simulink model "TrajGen"  (R2015a)
settings: Solver=ode45  StartTime=0.0  StopTime=10.0  RelTol=1e-3
values from neighbouring files (symbols this model uses):
  hf = 0    [ConvertToTimeseries.m]    (also in createTrajectories.m = -90)
  hi = 0    [ConvertToTimeseries.m]    (also in createTrajectories.m = 20)
  l = 10    [ConvertToTimeseries.m]    (also in createTrajectories.m = 3)
  xf = 63.37    [ConvertToTimeseries.m]    (also in createTrajectories.m = -5; genTraj.m = FC(1:3))
  xi = -10.89    [ConvertToTimeseries.m]    (also in createTrajectories.m = -6; genTraj.m = IC(1:3))
  yf = 48.737    [ConvertToTimeseries.m]    (also in createTrajectories.m = -6)
  yi = 48.737    [ConvertToTimeseries.m]    (also in createTrajectories.m = 2)
  zf = 2.33    [ConvertToTimeseries.m]    (also in createTrajectories.m = 2)
  zi = 2.33    [ConvertToTimeseries.m]    (also in createTrajectories.m = 2)
libraries: simulink x1
settings Model: CovSFcnEnable=off  Creator=cichell2  LastModifiedBy=marinho
settings DebuggingCC: SolverPrmCheckMsg=warning

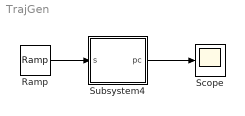
== system TrajGen ==
  Ramp : simulink/Sources/Ramp  slope=0.1  start=0  X0=0
  Scope : Scope
      settings: SaveName=Trajectory
  Subsystem4 : Subsystem
  wires:
  Ramp/1 -> Subsystem4/1(s)
  Subsystem4/1(pc) -> Scope/1

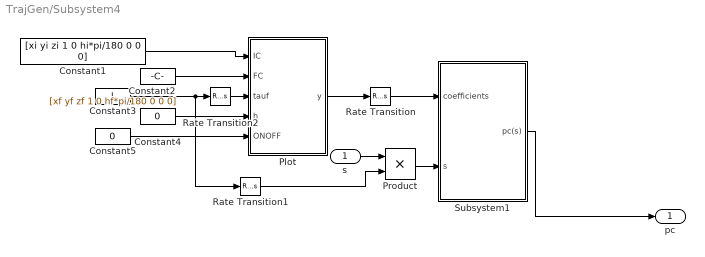
== system TrajGen/Subsystem4 ==
  s : Inport
  Constant1 : Constant  Value=[xi yi zi 1 0 hi*pi/180 0 0 0]
  Constant2 : Constant  Value=[xf yf zf 1 0 hf*pi/180 0 0 0]
  Constant3 : Constant  Value=l
  Constant4 : Constant  Value=0
  Constant5 : Constant  Value=0
  Plot : MATLAB Function  TreatAsAtomicUnit=on  SystemSampleTime=0.1
  Product : Product  RndMeth=Zero
  Rate Transition : RateTransition  OutPortSampleTime=0.01
  Rate Transition1 : RateTransition  OutPortSampleTimeOpt=Inherit  OutPortSampleTime=0.1
  Rate Transition2 : RateTransition  OutPortSampleTimeOpt=Inherit  OutPortSampleTime=0.1
  Subsystem1 : Subsystem
  pc : Outport
  wires:
  Plot/1(y) -> Rate Transition/1
  Constant1/1 -> Plot/1(IC)
  Constant2/1 -> Plot/2(FC)
  Constant3/1 -> Rate Transition1/1, Rate Transition2/1
  Constant4/1 -> Plot/4(h)
  Constant5/1 -> Plot/5(ONOFF)
  Subsystem1/1(pc(s)) -> pc/1
  Rate Transition/1 -> Subsystem1/1(coefficients)
  Product/1 -> Subsystem1/2(s)
  s/1 -> Product/1
  Rate Transition1/1 -> Product/2
  Rate Transition2/1 -> Plot/3(tauf)

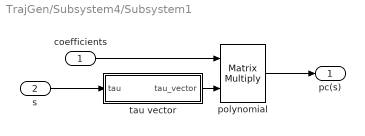
== system TrajGen/Subsystem4/Subsystem1 ==
  coefficients : Inport
  s : Inport  Port=2
  polynomial : Product  Multiplication=Matrix(*)  SaturateOnIntegerOverflow=on  OutDataTypeStr=Inherit: Same as first input
  tau vector : Subsystem
  pc(s) : Outport
  wires:
  polynomial/1 -> pc(s)/1
  coefficients/1 -> polynomial/1
  s/1 -> tau vector/1(tau)
  tau vector/1(tau_vector) -> polynomial/2

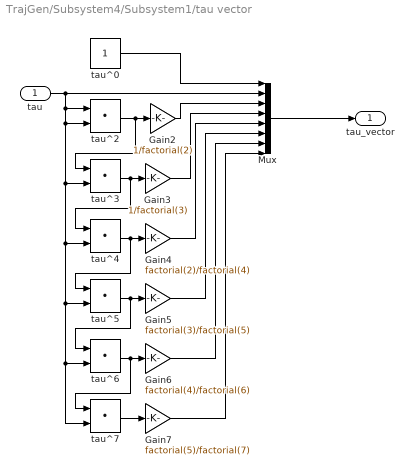
== system TrajGen/Subsystem4/Subsystem1/tau vector ==
  tau : Inport
  Gain2 : Gain  Gain=1/factorial(2)  SaturateOnIntegerOverflow=on  OutDataTypeStr=Inherit: Same as input  ParamDataTypeStr=Inherit: Same as input
  Gain3 : Gain  Gain=1/factorial(3)  SaturateOnIntegerOverflow=on  OutDataTypeStr=Inherit: Same as input  ParamDataTypeStr=Inherit: Same as input
  Gain4 : Gain  Gain=factorial(2)/factorial(4)  SaturateOnIntegerOverflow=on  OutDataTypeStr=Inherit: Same as input  ParamDataTypeStr=Inherit: Same as input
  Gain5 : Gain  Gain=factorial(3)/factorial(5)  SaturateOnIntegerOverflow=on  OutDataTypeStr=Inherit: Same as input  ParamDataTypeStr=Inherit: Same as input
  Gain6 : Gain  Gain=factorial(4)/factorial(6)  SaturateOnIntegerOverflow=on  OutDataTypeStr=Inherit: Same as input  ParamDataTypeStr=Inherit: Same as input
  Gain7 : Gain  Gain=factorial(5)/factorial(7)  SaturateOnIntegerOverflow=on  OutDataTypeStr=Inherit: Same as input  ParamDataTypeStr=Inherit: Same as input
  Mux : Mux  Inputs=8
  tau^0 : Constant
  tau^{2..7} (6 alike) : DotProduct  InputSameDT=on  OutDataTypeStr=Inherit: Inherit via internal rule
  tau_vector : Outport
  wires:
  tau^6/1 -> tau^7/1, Gain6/1
  tau^7/1 -> Gain7/1
  Gain7/1 -> Mux/8
  Gain6/1 -> Mux/7
  Gain4/1 -> Mux/5
  Gain5/1 -> Mux/6
  tau^5/1 -> tau^6/1, Gain5/1
  Gain2/1 -> Mux/3
  Gain3/1 -> Mux/4
  tau^4/1 -> tau^5/1, Gain4/1
  tau^2/1 -> Gain2/1, tau^3/1
  tau^0/1 -> Mux/1
  tau^3/1 -> Gain3/1, tau^4/1
  tau/1 -> tau^7/2, tau^6/2, tau^5/2, tau^4/2, tau^3/2, tau^2/2, tau^2/1, Mux/2
  Mux/1 -> tau_vector/1

== matlab function TrajGen/Subsystem4/Plot ==
  settings: fimath=|
      | fimath(...
      | 'RoundMode', 'floor',...
      | 'OverflowMode', 'wrap',...
      | 'ProductMode', 'KeepLSB', 'ProductWordLength', 32,...
      | 'SumMode', 'KeepLSB', 'SumWordLength', 32,...
      | 'CastBeforeSum', false)
  data: IC input; FC input; tauf input; y output; h input; ONOFF input
function y = plot3D(IC,FC,tauf,h,ONOFF)

%% Interface
%   IC,FC   - terminal conditions
%   tauf    - length of the dimensionless arc
%   h       - graphics handle:: trajectory plot
% Generated trajectory
%% Initialization and mappingof terminal conditions
% IC-"i" d/dt-"dt"  d/dtau-"p"
%
d2r=1;
xi=IC(1:3);
Vi=IC(4);
teti=d2r*IC(5);psi=d2r*IC(6);
Axi=IC(7);
tetidt=d2r*IC(8);psidt=d2r*IC(9);
% TeminalC-"f" d/dt-"dt"  d/dtau-"p"
%
xf=FC(1:3);
Vf=FC(4);
tetf=d2r*FC(5);psif=d2r*FC(6);
Axf=FC(7);
tetfdt=d2r*FC(8);psifdt=d2r*FC(9);
%% Derivatives at IC
%
xidt=[Vi*cos(teti)*cos(psi);...
    Vi*cos(teti)*sin(psi);...
    Vi*sin(teti)];
xip=xidt/Vi;
xi2dt=xip*Axi+Vi*[-tetidt*sin(teti)*cos(psi)-psidt*cos(teti)*sin(psi);...
    -tetidt*sin(teti)*sin(psi)+psidt*cos(teti)*cos(psi);...
    tetidt*cos(teti)];
xi2p=(xi2dt-xidt*Axi/Vi)/Vi^2;
xi3p=[0; 0; 0];
%% Derivatives at FC
%
xfdt=[Vf*cos(tetf)*cos(psif);...
    Vf*cos(tetf)*sin(psif);...
    Vf*sin(tetf)];
xfp=xfdt/Vf;
xf2dt=xfp*Axf+Vf*[-tetfdt*sin(tetf)*cos(psif)-psifdt*cos(tetf)*sin(psif);...
    -tetfdt*sin(tetf)*sin(psif)+psifdt*cos(tetf)*cos(psif);...
    tetfdt*cos(tetf)];
xf2p=(xf2dt-xfdt*Axf/Vf)/Vf^2;
xf3p=[0; 0; 0];
%% Polynomial coefficients of 7th order polinomial

 a0 = xi; a1 = xip; a2 = xi2p; a3 = xi3p;
 a4 = -(2*xf3p+8*xi3p)/tauf + (30*xf2p - 60*xi2p)/(tauf^2) - (180*xfp + 240*xip)/(tauf^3) + 420*(xf-xi)/(tauf^4);
 a5 = (10*xf3p+20*xi3p)/(tauf^2) - (140*xf2p - 200*xi2p)/(tauf^3) + (780*xfp + 900*xip)/(tauf^4) - 1680*(xf-xi)/(tauf^5);
 a6 = -(15*xf3p+20*xi3p)/(tauf^3) + (195*xf2p - 225*xi2p)/(tauf^4) - (1020*xfp + 1080*xip)/(tauf^5) + 2100*(xf-xi)/(tauf^6);
 a7 = 7*(xf3p+xi3p)/(tauf^4) - 84*(xf2p - xi2p)/(tauf^5) + 420*(xfp + xip)/(tauf^6) - 840*(xf-xi)/(tauf^7);
 a = [a0 a1 a2 a3 a4 a5 a6 a7];
 %% Numerical run along the trajectory
 tau=0;
 S=eye(3,100);
 for i=0:99
     tau=tau+tauf/100;
     %%Tau_vector as a function of variable tau==position along the dimensionless path
     tauvector = [1 tau tau^2/factorial(2) tau^3/factorial(3) tau^4*factorial(2)/factorial(4) tau^5*factorial(3)/factorial(5) tau^6*factorial(4)/factorial(6) ...
         tau^7*factorial(5)/factorial(7)]';
     %% Get trajectory
         x=a*tauvector;
     S(1,i+1)=x(1,1);
     S(2,i+1)=x(2,1);
     S(3,i+1)=x(3,1);
 end
% 
y=a;
